simulink model "Komar"  (R2014b)
settings: Solver=ode45  StartTime=0.0  StopTime=10  RelTol=1e-4
values from neighbouring files (symbols this model uses):
  J = 0.0421    [code.m]
  ki1 = 2000    [code.m]
  kii = ki*ki/2    (= 2205000)    [code.m]
  km = 3*psipm*pn/2    (= 0.813)    [code.m]
  kw = 300    [code.m]
  kwi = kw*kw/2    (= 45000)    [code.m]
  L = 180*10^(-6)    (= 0.00018)    [code.m]
  mu = km/J    (= 19.3111638955)    [code.m]
  pn = 10    [code.m]
  psipm = 0.0542    [code.m]
  R = 18*10^(-3)    (= 0.018)    [code.m]
undefined symbols (not defined in the file): t_con, tramp, Wref
settings Model: Creator=Юрій  LastModifiedBy=draga

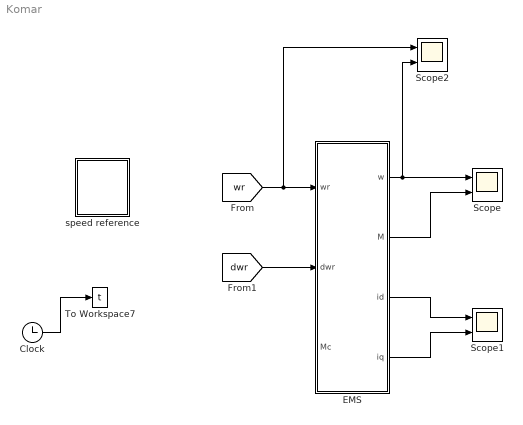
== system Komar ==
  Clock : Clock
  EMS : Subsystem
  Scope : Scope  NumInputPorts=2
      settings: YMin=0.912~149.15  YMax=1.008~164.85  SaveName=ScopeData7
  Scope1 : Scope  NumInputPorts=2
      settings: YMin=0.912~149.15  YMax=1.008~164.85
  Scope2 : Scope  NumInputPorts=2
      settings: YMin=0.912~149.15  YMax=1.008~164.85
  To Workspace7 : ToWorkspace  VariableName=t  SampleTime=-1
  speed reference : Subsystem  mask{wrmax=Wref, ta=tramp, ka=0.1, tcon=t_con, tex=1}
      mask prompts: wrmax "Speed value"; ta "Ramp time"; ka "Coef. smooth"; tcon "Const spped time"; tex "Excitation time"
  wires:
  Clock/1 -> To Workspace7/1
  [dwr] -> EMS/2(dwr)
  [wr] -> Scope2/1, EMS/1(wr)
  EMS/1(w) -> Scope2/2, Scope/1
  EMS/2(M) -> Scope/2
  EMS/3(id) -> Scope1/1
  EMS/4(iq) -> Scope1/2

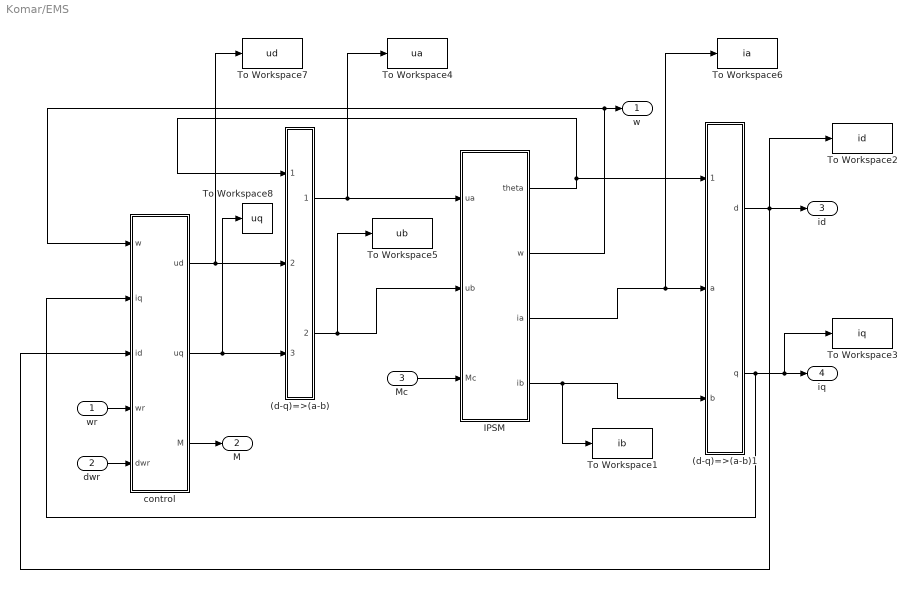
== system Komar/EMS ==
  wr : Inport
  dwr : Inport  Port=2
  Mc : Inport  Port=3
  (d-q)=>(a-b) : Subsystem
  (d-q)=>(a-b)1 : Subsystem
  IPSM : Subsystem
  To Workspace1 : ToWorkspace  VariableName=ib  SampleTime=-1
  To Workspace2 : ToWorkspace  VariableName=id  SampleTime=-1
  To Workspace3 : ToWorkspace  VariableName=iq  SampleTime=-1
  To Workspace4 : ToWorkspace  VariableName=ua  SampleTime=-1
  To Workspace5 : ToWorkspace  VariableName=ub  SampleTime=-1
  To Workspace6 : ToWorkspace  VariableName=ia  SampleTime=-1
  To Workspace7 : ToWorkspace  VariableName=ud  SampleTime=-1
  To Workspace8 : ToWorkspace  VariableName=uq  SampleTime=-1
  control : Subsystem
  w : Outport
  M : Outport  Port=2
  id : Outport  Port=3
  iq : Outport  Port=4
  wires:
  control/1(ud) -> To Workspace7/1, (d-q)=>(a-b)/2(d)
  Mc/1 -> IPSM/3(Mc)
  wr/1 -> control/4(wr)
  (d-q)=>(a-b)1/1(d) -> To Workspace2/1, id/1, control/3(id)
  (d-q)=>(a-b)1/2(q) -> To Workspace3/1, iq/1, control/2(iq)
  control/2(uq) -> To Workspace8/1, (d-q)=>(a-b)/3(q)
  IPSM/2(w) -> control/1(w), w/1
  IPSM/3(ia) -> To Workspace6/1, (d-q)=>(a-b)1/2(a)
  dwr/1 -> control/5(dwr)
  control/3("M ") -> M/1
  IPSM/1("theta ") -> (d-q)=>(a-b)/1("theta "), (d-q)=>(a-b)1/1("theta ")
  IPSM/4(ib) -> To Workspace1/1, (d-q)=>(a-b)1/3(b)
  (d-q)=>(a-b)/1(a) -> To Workspace4/1, IPSM/1(ua)
  (d-q)=>(a-b)/2(b) -> To Workspace5/1, IPSM/2(ub)

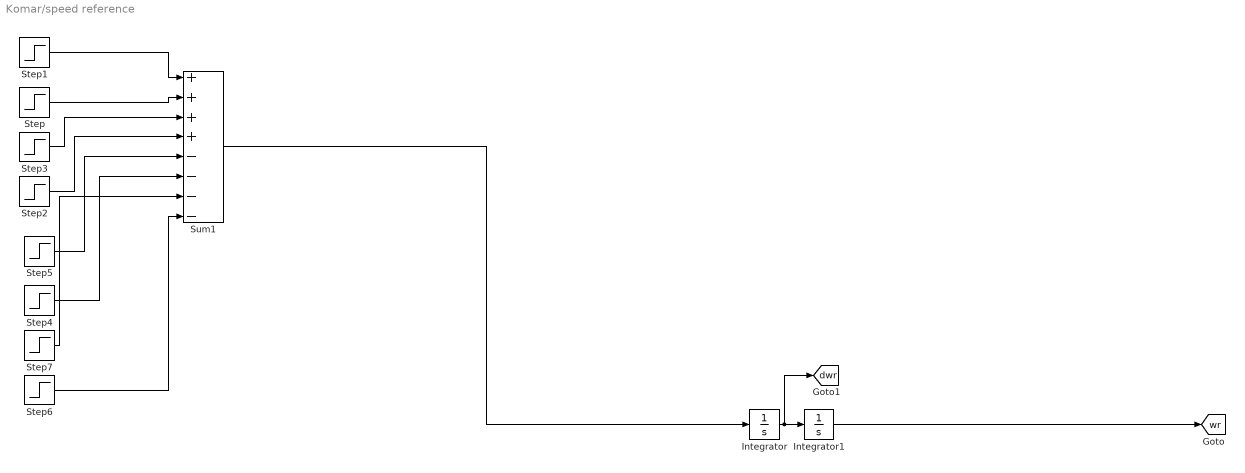
== system Komar/speed reference ==
  Integrator : Integrator
  Integrator1 : Integrator
  Step : Step  Time=tex+ta*ka  After=-wrmax/(ka*ta*ka*ta+ka*ta*(ta-2*ka*ta))
  Step1 : Step  Time=tex  After=wrmax/(ka*ta*ka*ta+ka*ta*(ta-2*ka*ta))
  Step2 : Step  Time=tex+ta  After=wrmax/(ka*ta*ka*ta+ka*ta*(ta-2*ka*ta))
  Step3 : Step  Time=tex+ta*ka+(ta-2*ta*ka)  After=-wrmax/(ka*ta*ka*ta+ka*ta*(ta-2*ka*ta))
  Step4 : Step  Time=tex+ta+tcon+ta*ka  After=-wrmax/(ka*ta*ka*ta+ka*ta*(ta-2*ka*ta))
  Step5 : Step  Time=tex+ta+tcon  After=wrmax/(ka*ta*ka*ta+ka*ta*(ta-2*ka*ta))
  Step6 : Step  Time=tex+ta+tcon+ta  After=wrmax/(ka*ta*ka*ta+ka*ta*(ta-2*ka*ta))
  Step7 : Step  Time=tex+ta+tcon+ta*ka+(ta-2*ta*ka)  After=-wrmax/(ka*ta*ka*ta+ka*ta*(ta-2*ka*ta))
  Sum1 : Sum  Inputs=++++----  SaturateOnIntegerOverflow=on  InputSameDT=on  OutDataTypeStr=Inherit: Same as first input
  tag scope: dwr=global, wr=global
  wires:
  Step1/1 -> Sum1/1
  Step/1 -> Sum1/2
  Step3/1 -> Sum1/3
  Step2/1 -> Sum1/4
  Step5/1 -> Sum1/5
  Integrator/1 -> Integrator1/1, [dwr]
  Step4/1 -> Sum1/6
  Step7/1 -> Sum1/7
  Step6/1 -> Sum1/8
  Sum1/1 -> Integrator/1
  Integrator1/1 -> [wr]

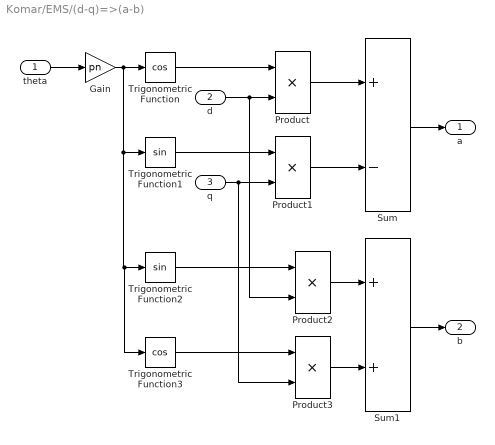
== system Komar/EMS/(d-q)=>(a-b) ==
  "theta " : Inport
  d : Inport  Port=2
  q : Inport  Port=3
  Gain : Gain  Gain=pn
  Product{,1..3} (4 alike) : Product
  Sum : Sum  Inputs=+-  SaturateOnIntegerOverflow=on  InputSameDT=on  OutDataTypeStr=Inherit: Same as first input
  Sum1 : Sum  SaturateOnIntegerOverflow=on  InputSameDT=on  OutDataTypeStr=Inherit: Same as first input
  Trigonometric Function : Trigonometry  Operator=cos
  Trigonometric Function1 : Trigonometry
  Trigonometric Function2 : Trigonometry
  Trigonometric Function3 : Trigonometry  Operator=cos
  a : Outport
  b : Outport  Port=2
  wires:
  Sum/1 -> a/1
  Trigonometric Function/1 -> Product/1
  Product/1 -> Sum/1
  Product1/1 -> Sum/2
  Trigonometric Function1/1 -> Product1/1
  q/1 -> Product3/2, Product1/2
  Sum1/1 -> b/1
  Product2/1 -> Sum1/1
  d/1 -> Product2/2, Product/2
  Product3/1 -> Sum1/2
  Trigonometric Function3/1 -> Product3/1
  Trigonometric Function2/1 -> Product2/1
  Gain/1 -> Trigonometric Function3/1, Trigonometric Function2/1, Trigonometric Function1/1, Trigonometric Function/1
  "theta "/1 -> Gain/1

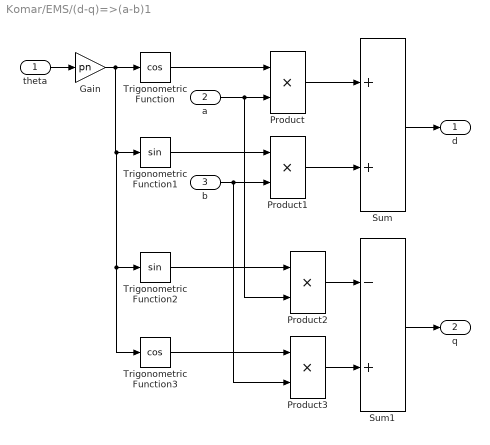
== system Komar/EMS/(d-q)=>(a-b)1 ==
  "theta " : Inport
  a : Inport  Port=2
  b : Inport  Port=3
  Gain : Gain  Gain=pn
  Product{,1..3} (4 alike) : Product
  Sum : Sum  SaturateOnIntegerOverflow=on  InputSameDT=on  OutDataTypeStr=Inherit: Same as first input
  Sum1 : Sum  Inputs=-+  SaturateOnIntegerOverflow=on  InputSameDT=on  OutDataTypeStr=Inherit: Same as first input
  Trigonometric Function : Trigonometry  Operator=cos
  Trigonometric Function1 : Trigonometry
  Trigonometric Function2 : Trigonometry
  Trigonometric Function3 : Trigonometry  Operator=cos
  d : Outport
  q : Outport  Port=2
  wires:
  Trigonometric Function2/1 -> Product2/1
  Trigonometric Function3/1 -> Product3/1
  Product3/1 -> Sum1/2
  a/1 -> Product/2, Product2/2
  Product2/1 -> Sum1/1
  Sum1/1 -> q/1
  b/1 -> Product1/2, Product3/2
  Trigonometric Function1/1 -> Product1/1
  Product1/1 -> Sum/2
  Product/1 -> Sum/1
  Trigonometric Function/1 -> Product/1
  Sum/1 -> d/1
  Gain/1 -> Trigonometric Function3/1, Trigonometric Function2/1, Trigonometric Function1/1, Trigonometric Function/1
  "theta "/1 -> Gain/1

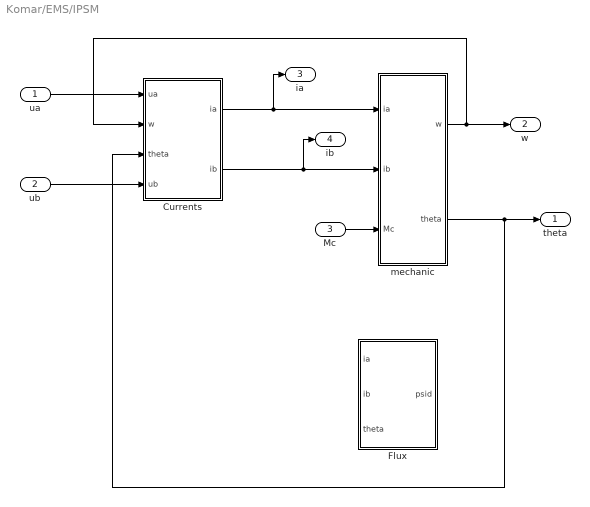
== system Komar/EMS/IPSM ==
  ua : Inport
  ub : Inport  Port=2
  Mc : Inport  Port=3
  Currents : Subsystem
  Flux : Subsystem
  mechanic : Subsystem
  "theta " : Outport
  w : Outport  Port=2
  ia : Outport  Port=3
  ib : Outport  Port=4
  wires:
  Currents/1(ia) -> mechanic/1(ia), ia/1
  Currents/2(ib) -> mechanic/2(ib), ib/1
  ua/1 -> Currents/1(ua)
  ub/1 -> Currents/4(ub)
  Mc/1 -> mechanic/3(Mc)
  mechanic/1(w) -> Currents/2(w), w/1
  mechanic/2(theta) -> "theta "/1, Currents/3(theta)

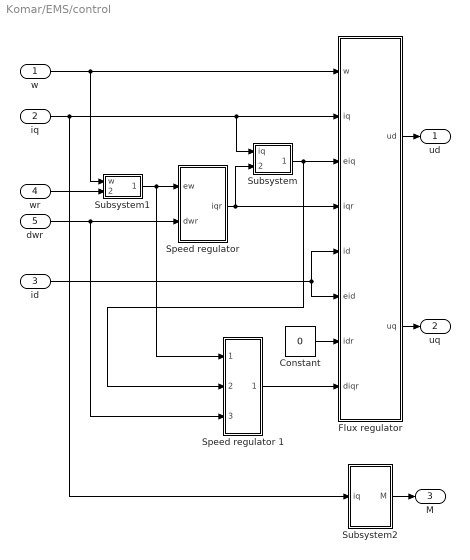
== system Komar/EMS/control ==
  w : Inport
  iq : Inport  Port=2
  id : Inport  Port=3
  wr : Inport  Port=4
  dwr : Inport  Port=5
  Constant : Constant  Value=0
  "Flux regulator " : Subsystem
  "Speed regulator " : Subsystem
  Speed regulator 1 : Subsystem
  Subsystem : Subsystem
  Subsystem1 : Subsystem
  Subsystem2 : Subsystem
  ud : Outport
  uq : Outport  Port=2
  "M " : Outport  Port=3
  wires:
  "Speed regulator "/1(iqr) -> Subsystem/2(iqr), "Flux regulator "/4("iqr ")
  "Flux regulator "/1(ud) -> ud/1
  "Flux regulator "/2("uq ") -> uq/1
  w/1 -> "Flux regulator "/1(w), Subsystem1/1(w)
  Constant/1 -> "Flux regulator "/7(idr)
  id/1 -> "Flux regulator "/5(id), "Flux regulator "/6(eid)
  dwr/1 -> Speed regulator 1/3(dwr), "Speed regulator "/2(dwr)
  iq/1 -> Subsystem2/1(iq), Subsystem/1(iq), "Flux regulator "/2(iq)
  Speed regulator 1/1(diqr) -> "Flux regulator "/8(diqr)
  Subsystem/1(eiq) -> "Flux regulator "/3("eiq "), Speed regulator 1/2(eiq)
  Subsystem1/1(ew) -> Speed regulator 1/1(ew), "Speed regulator "/1(ew)
  wr/1 -> Subsystem1/2(wr)
  Subsystem2/1("M ") -> "M "/1

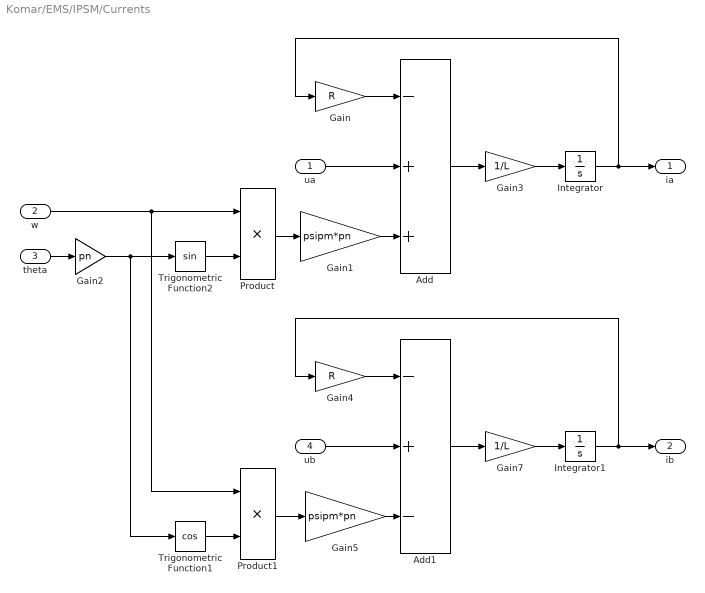
== system Komar/EMS/IPSM/Currents ==
  ua : Inport
  w : Inport  Port=2
  theta : Inport  Port=3
  ub : Inport  Port=4
  Add : Sum  Inputs=-++
  Add1 : Sum  Inputs=-+-
  Gain : Gain  Gain=R
  Gain1 : Gain  Gain=psipm*pn
  Gain2 : Gain  Gain=pn
  Gain3 : Gain  Gain=1/L
  Gain4 : Gain  Gain=R
  Gain5 : Gain  Gain=psipm*pn
  Gain7 : Gain  Gain=1/L
  Integrator : Integrator
  Integrator1 : Integrator
  Product : Product
  Product1 : Product
  Trigonometric Function1 : Trigonometry  Operator=cos
  Trigonometric Function2 : Trigonometry
  ia : Outport
  ib : Outport  Port=2
  wires:
  Gain2/1 -> Trigonometric Function2/1, Trigonometric Function1/1
  Add/1 -> Gain3/1
  Gain3/1 -> Integrator/1
  Product/1 -> Gain1/1
  Gain1/1 -> Add/3
  ua/1 -> Add/2
  Integrator/1 -> ia/1, Gain/1
  Trigonometric Function1/1 -> Product1/2
  Gain5/1 -> Add1/3
  ub/1 -> Add1/2
  Add1/1 -> Gain7/1
  Product1/1 -> Gain5/1
  Gain7/1 -> Integrator1/1
  Gain4/1 -> Add1/1
  Integrator1/1 -> ib/1, Gain4/1
  Gain/1 -> Add/1
  w/1 -> Product1/1, Product/1
  theta/1 -> Gain2/1
  Trigonometric Function2/1 -> Product/2

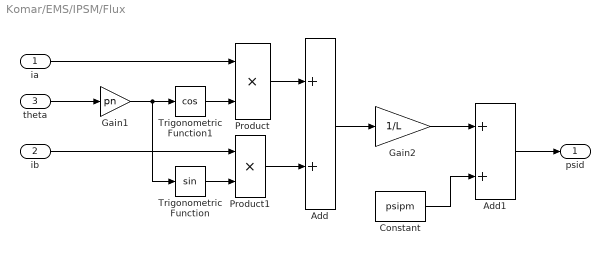
== system Komar/EMS/IPSM/Flux ==
  ia : Inport
  ib : Inport  Port=2
  theta : Inport  Port=3
  Add : Sum
  Add1 : Sum
  Constant : Constant  Value=psipm
  Gain1 : Gain  Gain=pn
  Gain2 : Gain  Gain=1/L
  Product : Product
  Product1 : Product
  Trigonometric Function : Trigonometry
  Trigonometric Function1 : Trigonometry  Operator=cos
  psid : Outport
  wires:
  theta/1 -> Gain1/1
  Product1/1 -> Add/2
  Add1/1 -> psid/1
  Trigonometric Function/1 -> Product1/2
  Gain1/1 -> Trigonometric Function/1, Trigonometric Function1/1
  ia/1 -> Product/1
  Trigonometric Function1/1 -> Product/2
  Product/1 -> Add/1
  ib/1 -> Product1/1
  Gain2/1 -> Add1/1
  Add/1 -> Gain2/1
  Constant/1 -> Add1/2

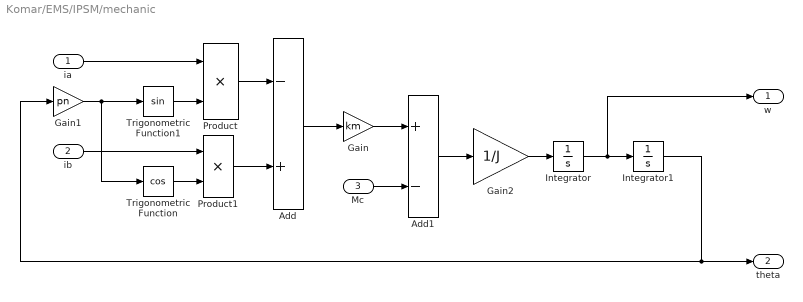
== system Komar/EMS/IPSM/mechanic ==
  ia : Inport
  ib : Inport  Port=2
  Mc : Inport  Port=3
  Add : Sum  Inputs=-+
  Add1 : Sum  Inputs=+-
  Gain : Gain  Gain=km
  Gain1 : Gain  Gain=pn
  Gain2 : Gain  Gain=1/J
  Integrator : Integrator  InitialCondition=0.001
  Integrator1 : Integrator
  Product : Product
  Product1 : Product
  Trigonometric Function : Trigonometry  Operator=cos
  Trigonometric Function1 : Trigonometry
  w : Outport
  theta : Outport  Port=2
  wires:
  Integrator/1 -> w/1, Integrator1/1
  Product/1 -> Add/1
  ib/1 -> Product1/1
  Add/1 -> Gain/1
  Trigonometric Function1/1 -> Product/2
  Trigonometric Function/1 -> Product1/2
  ia/1 -> Product/1
  Integrator1/1 -> theta/1, Gain1/1
  Product1/1 -> Add/2
  Gain/1 -> Add1/1
  Mc/1 -> Add1/2
  Add1/1 -> Gain2/1
  Gain2/1 -> Integrator/1
  Gain1/1 -> Trigonometric Function/1, Trigonometric Function1/1

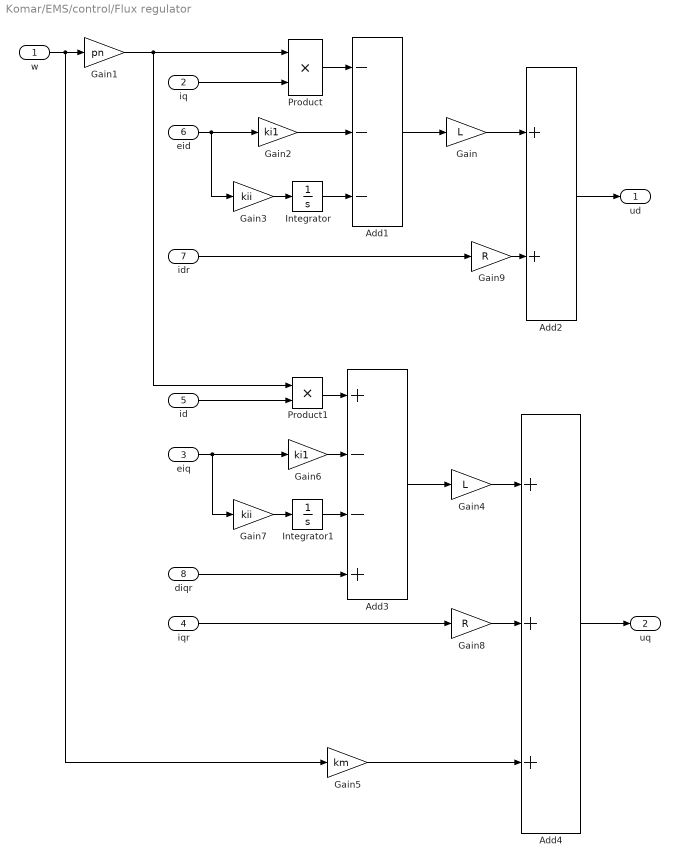
== system Komar/EMS/control/Flux regulator  ==
  w : Inport
  iq : Inport  Port=2
  "eiq " : Inport  Port=3
  "iqr " : Inport  Port=4
  id : Inport  Port=5
  eid : Inport  Port=6
  idr : Inport  Port=7
  diqr : Inport  Port=8
  Add1 : Sum  Inputs=---
  Add2 : Sum
  Add3 : Sum  Inputs=+--+
  Add4 : Sum  Inputs=+++
  Gain : Gain  Gain=L
  Gain1 : Gain  Gain=pn
  Gain2 : Gain  Gain=ki1
  Gain3 : Gain  Gain=kii
  Gain4 : Gain  Gain=L
  Gain5 : Gain  Gain=km
  Gain6 : Gain  Gain=ki1
  Gain7 : Gain  Gain=kii
  Gain8 : Gain  Gain=R
  Gain9 : Gain  Gain=R
  Integrator : Integrator
  Integrator1 : Integrator
  Product : Product
  Product1 : Product
  ud : Outport
  "uq " : Outport  Port=2
  wires:
  Add1/1 -> Gain/1
  Gain/1 -> Add2/1
  Product/1 -> Add1/1
  Gain1/1 -> Product1/1, Product/1
  iq/1 -> Product/2
  eid/1 -> Gain3/1, Gain2/1
  Gain3/1 -> Integrator/1
  Integrator/1 -> Add1/3
  Add2/1 -> ud/1
  Add3/1 -> Gain4/1
  Gain4/1 -> Add4/1
  Product1/1 -> Add3/1
  w/1 -> Gain5/1, Gain1/1
  id/1 -> Product1/2
  Gain7/1 -> Integrator1/1
  Add4/1 -> "uq "/1
  Gain8/1 -> Add4/2
  "iqr "/1 -> Gain8/1
  "eiq "/1 -> Gain7/1, Gain6/1
  Gain2/1 -> Add1/2
  Gain6/1 -> Add3/2
  Integrator1/1 -> Add3/3
  idr/1 -> Gain9/1
  Gain9/1 -> Add2/2
  Gain5/1 -> Add4/3
  diqr/1 -> Add3/4

== system Komar/EMS/control/Speed regulator  ==
  ew : Inport
  dwr : Inport  Port=2
  Add : Sum  Inputs=--+
  Gain : Gain  Gain=1/mu
  Gain1 : Gain  Gain=kwi
  Gain2 : Gain  Gain=kw
  Integrator : Integrator
  iqr : Outport
  wires:
  dwr/1 -> Add/3
  Gain2/1 -> Add/2
  Integrator/1 -> Add/1
  Gain1/1 -> Integrator/1
  Gain/1 -> iqr/1
  Add/1 -> Gain/1
  ew/1 -> Gain1/1, Gain2/1

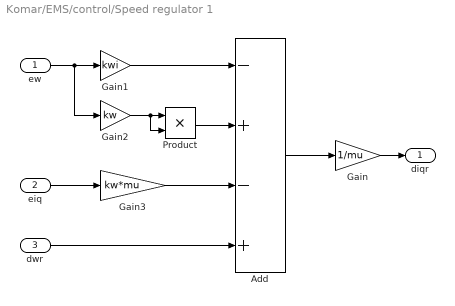
== system Komar/EMS/control/Speed regulator 1 ==
  ew : Inport
  eiq : Inport  Port=2
  dwr : Inport  Port=3
  Add : Sum  Inputs=-+-+
  Gain : Gain  Gain=1/mu
  Gain1 : Gain  Gain=kwi
  Gain2 : Gain  Gain=kw
  Gain3 : Gain  Gain=kw*mu
  Product : Product
  diqr : Outport
  wires:
  ew/1 -> Gain2/1, Gain1/1
  Add/1 -> Gain/1
  Gain/1 -> diqr/1
  Gain1/1 -> Add/1
  Product/1 -> Add/2
  Gain2/1 -> Product/2, Product/1
  dwr/1 -> Add/4
  eiq/1 -> Gain3/1
  Gain3/1 -> Add/3

== system Komar/EMS/control/Subsystem ==
  iq : Inport
  iqr : Inport  Port=2
  Add : Sum  Inputs=+-
  eiq : Outport
  wires:
  iq/1 -> Add/1
  iqr/1 -> Add/2
  Add/1 -> eiq/1

== system Komar/EMS/control/Subsystem1 ==
  w : Inport
  wr : Inport  Port=2
  Add1 : Sum  Inputs=+-
  ew : Outport
  wires:
  w/1 -> Add1/1
  Add1/1 -> ew/1
  wr/1 -> Add1/2

== system Komar/EMS/control/Subsystem2 ==
  iq : Inport
  Constant1 : Constant  Value=km
  Product2 : Product
  "M " : Outport
  wires:
  Constant1/1 -> Product2/1
  Product2/1 -> "M "/1
  iq/1 -> Product2/2
